simulink model "gazeboExampleParamServer"  (R2017b)
settings: Solver=FixedStepDiscrete  StartTime=0.0  StopTime=inf  FixedStep=params.Ts  RelTol=1e-3  EnableMultiTasking=on
PreLoadFcn:
  | params = controlParamsGazebo;
  | 
  | rosshutdown;
  | loadIpAddresses;
  | rosinit(gazeboIp);
  | 
  | % Initialize ROS parameters
  | rosparam('set','/gains/linear',params.linVelGain);
  | rosparam('set','/gains/angular',params.angVelGain);
model workspace (MAT data in the model file):
  SL_ROS_VariableLengthArrays_MaxSizes.CommonInfo.ArrayTruncateAction = 'EmitWarning'
  SL_ROS_VariableLengthArrays_MaxSizes.MsgTypeMap = containers.Map
  SL_ROS_VariableLengthArrays_MaxSizes.MsgTypeMap.serialization.keys = {'sensor_msgs/Image'}
  SL_ROS_VariableLengthArrays_MaxSizes.MsgTypeMap.serialization.values{1}(1).PropertyName = 'Data'
  SL_ROS_VariableLengthArrays_MaxSizes.MsgTypeMap.serialization.values{1}(1).DataType = 'uint8'
  SL_ROS_VariableLengthArrays_MaxSizes.MsgTypeMap.serialization.values{1}(1).MaxLength = 921600
  SL_ROS_VariableLengthArrays_MaxSizes.MsgTypeMap.serialization.values{1}(2).PropertyName = 'Encoding'
  SL_ROS_VariableLengthArrays_MaxSizes.MsgTypeMap.serialization.values{1}(2).DataType = 'uint8'
  SL_ROS_VariableLengthArrays_MaxSizes.MsgTypeMap.serialization.values{1}(2).MaxLength = 128
  SL_ROS_VariableLengthArrays_MaxSizes.MsgTypeMap.serialization.uniformity = 0
  SL_ROS_VariableLengthArrays_MaxSizes.MsgTypeMap.serialization.keyType = 'char'
  SL_ROS_VariableLengthArrays_MaxSizes.MsgTypeMap.serialization.valueType = 'any'
undefined symbols (not defined in the file): Angular, Linear
libraries: robotlib x6, visiontextngfix x1, controlLib x1, visionsinks x1
settings Model: Creator=scastro  LastModifiedBy=scastro
settings SolverCC: PositivePriorityOrder=on
settings OptimizationCC: PassReuseOutputArgsAs=Individual arguments  MaxStackSize=64
settings DebuggingCC: ParameterTunabilityLossMsg=error
settings HardwareCC: ProdBitPerLong=64  ProdHWDeviceType=Intel->x86-64 (Linux 64)
settings RTWCC: SystemTargetFile=ert.tlc  HardwareBoard=Robot Operating System (ROS)  TemplateMakefile=ert_default_tmf  GenerateReport=on  Toolchain=Catkin  IncludeHyperlinkInReport=on  LaunchReport=on  TargetLang=C++  GenerateTraceInfo=on  GenerateTraceReport=on  GenerateTraceReportSl=on  GenerateTraceReportSf=on  GenerateTraceReportEml=on
settings CodeAppCC: ForceParamTrailComments=on  IgnoreCustomStorageClasses=off  OperatorAnnotations=on  SimulinkDataObjDesc=on  SFDataObjDesc=on  MATLABFcnDesc=on  InsertBlockDesc=on  StateflowObjectComments=on  MATLABSourceComments=on
settings ERTTargetCC: SupportVariableSizeSignals=on

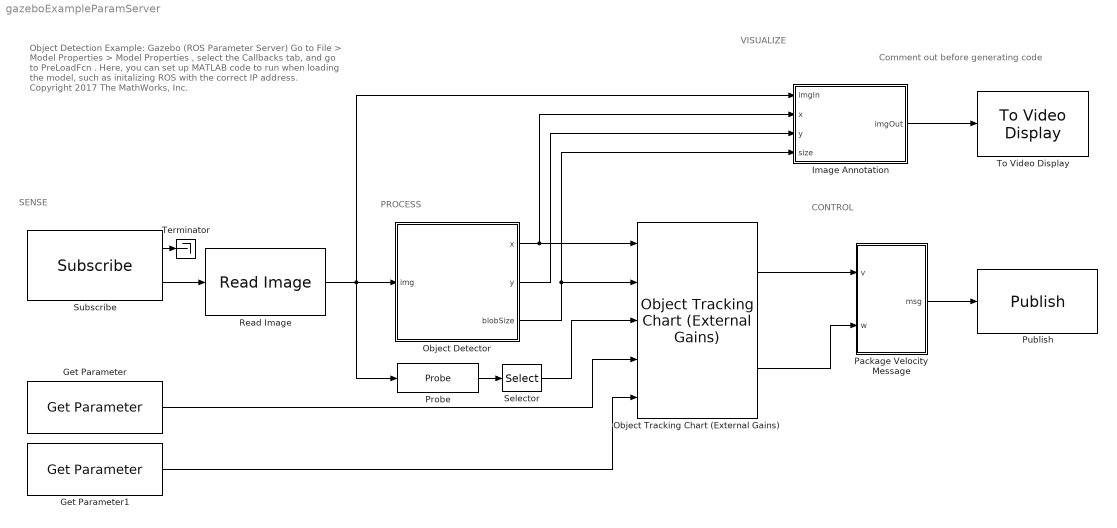
== system gazeboExampleParamServer ==
  note: CONTROL
  note: PROCESS
  note: SENSE
  note: Object Detection Example:
      | Gazebo (ROS Parameter Server)
      |
      | Go to File > Model Properties > Model Properties , select the Callbacks tab, and go to PreLoadFcn . Here, you can set up MATLAB code to run when loading the model, such as initalizing ROS with the correct IP address.
      |
      | Copyright 2017 The MathWorks, Inc.
  note: Comment out before generating code
  note: VISUALIZE
  Get Parameter : robotlib/Get Parameter  SourceLibraryInfo=This block requires Robotics System Toolbox  ParameterSource=Select from ROS network  ParameterName=/gains/linear  ParameterType=double  ParameterMaxArrayLength=16  ParameterInitialValue=0  SampleTime=-1  ShowErrorCodeOutput=off  ModelName=gazeboExampleParamServer  BlockId=ParamGet_gazeboExampleParamServer_194
      settings: SourceProductName=Robotics System Toolbox  SourceProductBaseCode=RO
  Get Parameter1 : robotlib/Get Parameter  SourceLibraryInfo=This block requires Robotics System Toolbox  ParameterSource=Select from ROS network  ParameterName=/gains/angular  ParameterType=double  ParameterMaxArrayLength=16  ParameterInitialValue=0  SampleTime=-1  ShowErrorCodeOutput=off  ModelName=gazeboExampleParamServer  BlockId=ParamGet_gazeboExampleParamServer_196
      settings: SourceProductName=Robotics System Toolbox  SourceProductBaseCode=RO
  Image Annotation : Subsystem
  Object Detector : MATLAB Function  TreatAsAtomicUnit=on
  Object Tracking Chart (External Gains) : controlLib/Object Tracking Chart  (External Gains)
  Package Velocity Message : Subsystem
  Probe : Probe  ProbeWidth=off  ProbeSampleTime=off  ProbeComplexSignal=off  ProbeSignalDimensions=on
  Publish : robotlib/Publish  SourceLibraryInfo=This block requires Robotics System Toolbox  topicSource=Select from ROS network  topic=/mobile_base/commands/velocity  messageType=geometry_msgs/Twist  messageQueueLength=1
      settings: SourceProductBaseCode=RO
  Read Image : robotlib/Read Image  SourceLibraryInfo=This block requires Robotics System Toolbox  MaximumImageSize=[480, 640]  ImageEncoding=rgb8  ShowAlphaOutput=off  ShowErrorCodeOutput=off  VariableSizeOutputs=off
      settings: SourceProductName=Robotics System Toolbox  SourceProductBaseCode=RO
  Selector : Selector  InputPortWidth=3  IndexOptions=Index vector (dialog)  Indices=2  OutputSizes=1
  Subscribe : robotlib/Subscribe  SourceLibraryInfo=This block requires Robotics System Toolbox  topicSource=Specify your own  topic=/camera/rgb/image_raw  messageType=sensor_msgs/Image  sampleTime=-1  messageQueueLength=1
      settings: SourceProductBaseCode=RO
  Terminator : Terminator
  To Video Display : visionsinks/To Video Display  windowSizeMode=Normal  openAtMdlStart=on  fullScreen=off  videoWindowX=964  videoWindowY=79  saveWindowSize=off  videoWindowWidth=725  videoWindowHeight=561  inputColorFormat=RGB  inputType=Obsolete  imagePorts=One multidimensional signal  OutputDevice=On-screen video monitor  dataOrg=Column-major  isWindowOpen=off
      settings: SourceProductName=Computer Vision System Toolbox
  wires:
  Object Detector/3(blobSize) -> Object Tracking Chart (External Gains)/2, Image Annotation/4(size)
  Probe/1 -> Selector/1
  Object Tracking Chart (External Gains)/1 -> Package Velocity Message/1(v)
  Object Tracking Chart (External Gains)/2 -> Package Velocity Message/2(w)
  Package Velocity Message/1(msg) -> Publish/1
  Subscribe/2 -> Read Image/1
  Subscribe/1 -> Terminator/1
  Get Parameter/1 -> Object Tracking Chart (External Gains)/4
  Get Parameter1/1 -> Object Tracking Chart (External Gains)/5
  Read Image/1 -> Image Annotation/1(imgIn), Probe/1, Object Detector/1(img)
  Object Detector/2(y) -> Image Annotation/3(y)
  Object Detector/1(x) -> Object Tracking Chart (External Gains)/1, Image Annotation/2(x)
  Image Annotation/1(imgOut) -> To Video Display/1
  Selector/1 -> Object Tracking Chart (External Gains)/3

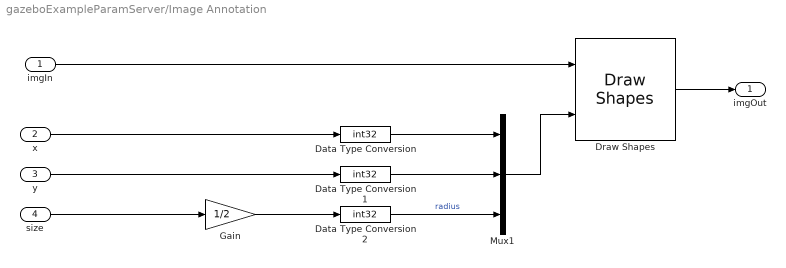
== system gazeboExampleParamServer/Image Annotation ==
  imgIn : Inport
  x : Inport  Port=2
  y : Inport  Port=3
  size : Inport  Port=4
  Data Type Conversion : DataTypeConversion  OutDataTypeStr=int32
  Data Type Conversion1 : DataTypeConversion  OutDataTypeStr=int32
  Data Type Conversion2 : DataTypeConversion  OutDataTypeStr=int32
  Draw Shapes : visiontextngfix/Draw Shapes  shape=Circles  fill=off  lineWidth=2  fillClrSource=Specify via dialog  display=User-specified value  intensity=200  color=[255 255 0]  opacity=0.6  viewport=Entire image  antialiasing=off  inType=Obsolete  imagePorts=One multidimensional signal  prodOutputMode=Binary point scaling  prodOutputWordLength=32  prodOutputFracLength=14  memoryMode=Specify word length  memoryWordLength=16  memoryFracLength=14  roundingMode=Floor  overflowMode=off
      settings: SourceProductName=Computer Vision System Toolbox
  Gain : Gain  Gain=1/2
  Mux1 : Mux  Inputs=3
  imgOut : Outport
  wires:
  y/1 -> Data Type Conversion1/1
  Data Type Conversion1/1 -> Mux1/2
  Data Type Conversion/1 -> Mux1/1
  x/1 -> Data Type Conversion/1
  imgIn/1 -> Draw Shapes/1
  Draw Shapes/1 -> imgOut/1
  Mux1/1 -> Draw Shapes/2
  Gain/1 -> Data Type Conversion2/1
  size/1 -> Gain/1
  Data Type Conversion2/1 -> Mux1/3  "radius"

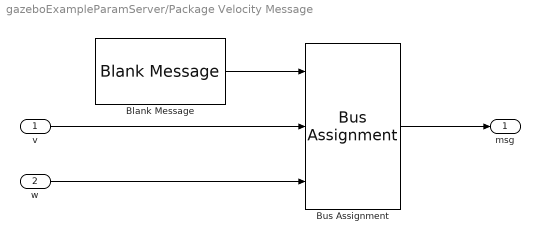
== system gazeboExampleParamServer/Package Velocity Message ==
  v : Inport
  w : Inport  Port=2
  Blank Message : robotlib/Blank Message  SourceLibraryInfo=This block requires Robotics System Toolbox  messageType=geometry_msgs/Twist  SampleTime=inf
      settings: SourceProductBaseCode=RO
  Bus Assignment : BusAssignment  AssignedSignals=Linear.X,Angular.Z
  msg : Outport
  wires:
  Blank Message/1 -> Bus Assignment/1
  Bus Assignment/1 -> msg/1
  w/1 -> Bus Assignment/3
  v/1 -> Bus Assignment/2

== matlab function gazeboExampleParamServer/Object Detector ==
  data: x output; img input; y output; blobSize output
function [x,y,blobSize] = CircleDetection(img)
    
    % Initialize outputs
    x = 0;
    y = 0;
    blobSize = 0;
    
    % Call external function
    resizeScale = 0.5;
    [x,y,blobSize] = detectCircle(img,resizeScale);

end
